simulink model "Bachelor_PanizEilkhani"  (R2020b)
settings: Solver=VariableStepAuto  StartTime=0.0  StopTime=80  RelTol=1e-3
libraries: simulink x3
settings Model: Creator=takro  LastModifiedBy=takro

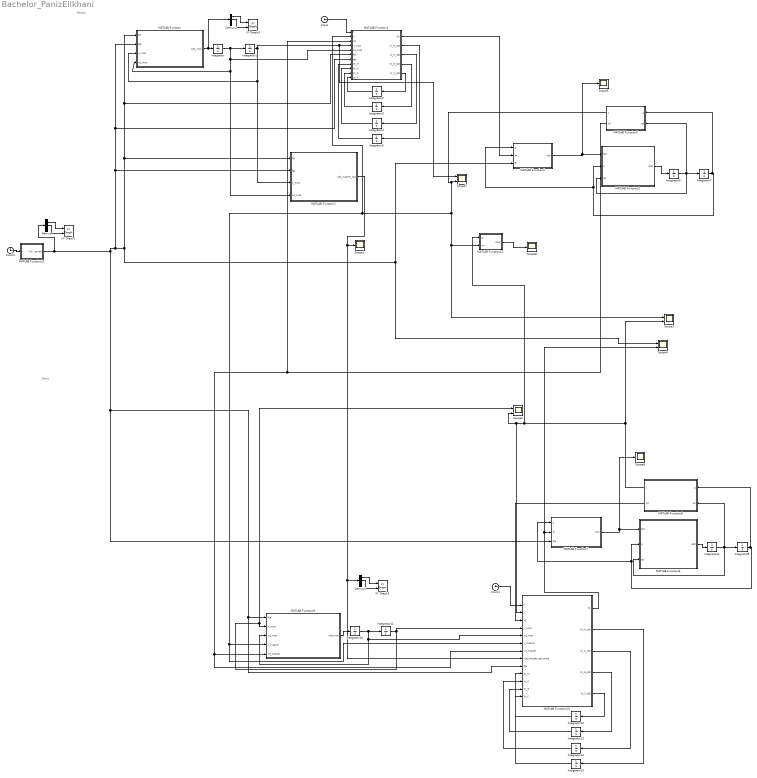
== system Bachelor_PanizEilkhani ==
  note: Master
  note: ُSlave
  Clock : Clock
  Clock1 : Clock
  Clock2 : Clock
  Demux : Demux  Outputs=3
  Demux1 : Demux  Outputs=3
  Demux2 : Demux  Outputs=3
  Integrator{,1,10..11} (4 alike) : Integrator  InitialCondition=[1 1 1]'*0
  Integrator{2..3,12..13} (4 alike) : Integrator  InitialCondition=ones(3, 3)
  Integrator{4..5,14..15} (4 alike) : Integrator  InitialCondition=ones(9, 3)
  Integrator{6..9} (4 alike) : Integrator  InitialCondition=[1 1 1]*0
  MATLAB Function : MATLAB Function  TreatAsAtomicUnit=on
  MATLAB Function1 : MATLAB Function  TreatAsAtomicUnit=on
  MATLAB Function10 : MATLAB Function  TreatAsAtomicUnit=on
  MATLAB Function11 : MATLAB Function  TreatAsAtomicUnit=on
  MATLAB Function12 : MATLAB Function  TreatAsAtomicUnit=on
  MATLAB Function2 : MATLAB Function  TreatAsAtomicUnit=on
  MATLAB Function3 : MATLAB Function  TreatAsAtomicUnit=on
  MATLAB Function4 : MATLAB Function  TreatAsAtomicUnit=on
  MATLAB Function5 : MATLAB Function  TreatAsAtomicUnit=on
  MATLAB Function6 : MATLAB Function  TreatAsAtomicUnit=on
  MATLAB Function7 : MATLAB Function  TreatAsAtomicUnit=on
  MATLAB Function8 : MATLAB Function  TreatAsAtomicUnit=on
  MATLAB Function9 : MATLAB Function  TreatAsAtomicUnit=on
  Scope{1,5..6,8} (4 alike) : Scope
  Scope{2..4,7} (4 alike) : Scope  NumInputPorts=2
  XY Graph1 : simulink/Sinks/XY Graph  xmin=-20  xmax=20  ymin=-20  ymax=20  st=0
  XY Graph2 : simulink/Sinks/XY Graph  xmin=-20  xmax=20  ymin=-20  ymax=20  st=0
  XY Graph3 : simulink/Sinks/XY Graph  xmin=-20  xmax=20  ymin=-20  ymax=20  st=0
  wires:
  Clock/1 -> MATLAB Function1/1(t)
  Integrator5/1 -> MATLAB Function1/8(W_M)
  MATLAB Function1/5(W_F_dot) -> Integrator2/1
  Integrator2/1 -> MATLAB Function1/11(W_F)
  MATLAB Function1/2(W_M_dot) -> Integrator5/1
  MATLAB Function1/3(W_C_dot) -> Integrator4/1
  Integrator/1 -> Integrator1/1, MATLAB Function1/5(xd_mod), MATLAB Function2/4(xd_mod), MATLAB Function/4(xd_mod)
  MATLAB Function1/4(W_G_dot) -> Integrator3/1
  Integrator4/1 -> MATLAB Function1/9(W_C)
  Integrator1/1 -> Scope7/1, MATLAB Function1/4(x_mod), MATLAB Function2/3(x_mod), MATLAB Function/3(x_mod)
  Integrator3/1 -> MATLAB Function1/10(W_G)
  MATLAB Function4/1(taw) -> Scope5/1, MATLAB Function3/1(taw)
  MATLAB Function3/1(qdd) -> Integrator6/1
  Integrator6/1 -> MATLAB Function5/2(qd), MATLAB Function3/3(qd), Integrator7/1
  MATLAB Function1/1(fm) -> MATLAB Function4/2(fm)
  Integrator7/1 -> MATLAB Function5/1(q), MATLAB Function4/1(q), MATLAB Function3/2(q)
  Integrator8/1 -> MATLAB Function8/2(qd), MATLAB Function6/3(qd), Integrator9/1
  MATLAB Function6/1(qdd) -> Integrator8/1
  Integrator9/1 -> MATLAB Function8/1(q), MATLAB Function7/1(q), MATLAB Function6/2(q)
  MATLAB Function7/1(taw) -> Scope6/1, MATLAB Function6/1(taw)
  MATLAB Function5/2(xd) -> MATLAB Function9/5(xd_master), MATLAB Function10/7(xd_master), MATLAB Function1/3(xd)
  Integrator12/1 -> MATLAB Function10/13(W_F)
  MATLAB Function10/2(W_M_dot) -> Integrator15/1
  MATLAB Function10/1(fs) -> Scope4/2, MATLAB Function7/2(fs)
  MATLAB Function10/5(W_F_dot) -> Integrator12/1
  Integrator11/1 -> MATLAB Function10/4(x_mod), Scope2/1, MATLAB Function9/2(x_mod)
  MATLAB Function8/2(xd) -> MATLAB Function10/3(xd)
  MATLAB Function2/1(xdd_master_hat) -> Demux1/1, MATLAB Function10/8(xdd_master_estimate), Scope1/1
  Integrator13/1 -> MATLAB Function10/12(W_G)
  Integrator15/1 -> MATLAB Function10/10(W_M)
  MATLAB Function10/3(W_C_dot) -> Integrator14/1
  Clock1/1 -> MATLAB Function10/1(t)
  Integrator14/1 -> MATLAB Function10/11(W_C)
  Integrator10/1 -> MATLAB Function10/5(xd_mod), MATLAB Function9/3(xd_mod), Integrator11/1
  MATLAB Function5/1(x) -> Scope7/2, MATLAB Function12/2(xm), Scope3/1, MATLAB Function10/6(x_master), MATLAB Function9/4(x_master), MATLAB Function1/2(x)
  MATLAB Function11/1(Xm_desired) -> Demux/1, MATLAB Function7/3(fpa), MATLAB Function10/9(fpa), MATLAB Function9/1(fpa), Scope4/1, MATLAB Function4/3(fh), MATLAB Function/1(fth), MATLAB Function1/6(fth), MATLAB Function2/1(fth), MATLAB Function/2(fpa), MATLAB Function1/7(fpa), MATLAB Function2/2(fpa)
  MATLAB Function9/1(xdd_mod) -> Integrator10/1
  MATLAB Function10/4(W_G_dot) -> Integrator13/1
  Clock2/1 -> MATLAB Function11/1(t)
  Demux/1 -> XY Graph2/1
  Demux/2 -> XY Graph2/2
  Demux1/2 -> XY Graph1/2
  Demux1/1 -> XY Graph1/1
  MATLAB Function8/1(x) -> Scope3/2, MATLAB Function12/1(xs), MATLAB Function10/2(x), Scope2/2
  MATLAB Function12/1(out3) -> Scope8/1
  Demux2/1 -> XY Graph3/1
  MATLAB Function/1(xdd_mod) -> Demux2/1, Integrator/1
  Demux2/2 -> XY Graph3/2

== matlab function Bachelor_PanizEilkhani/MATLAB Function10 ==
  data: t input; x input; fs output; xd input; x_mod input; xd_mod input; x_master input; xd_master input; xdd_master_estimate input; fpa input; W_M input; W_C input; W_G input; W_M_dot output; W_C_dot output; W_G_dot output; W_F_dot output; W_F input
function [fs, W_M_dot, W_C_dot, W_G_dot, W_F_dot] = slave_controller(t, x, xd, x_mod, xd_mod, x_master, xd_master, xdd_master_estimate, fpa, W_M, W_C, W_G, W_F)

landa1 = 1;
landa2 = 3;
landa3 = 0;
kp = 1;
m = eye(3)*15;
c = eye(3)*2500;
k = eye(3)*14000;
invm = inv(m);

fn = 5;
    
zz = [1; sin(fn*t); sin(2*fn*t)];
Z_M = [zz zeros(3, 2) ; zeros(3, 1) zz zeros(3, 1); zeros(3, 2) zz];
Z_C = Z_M;
Z_G = zz; % note G is not like above ones
Z_F = zz; % note F is not like above ones

M_hat = W_M'*Z_M;
C_hat = W_C'*Z_C;
G_hat = W_G'*Z_G;
F_hat = W_F'*Z_F;

Q_M = eye(9)*100;
Q_C = eye(9)*100;
Q_G = eye(3)*100; % note the dimention
Q_F = eye(3)*100; % note the dimention

R = kp*xdd_master_estimate - (invm*c)*(xd-kp*xd_master) - (invm*k)*(x - kp*x_master) + invm*(-fpa) + (landa3^2)*(x-x_mod);
S = (xd-xd_mod) + landa1*(x-x_mod);

W_M_dot = -pinv(Q_M)*Z_M*R*S';
W_C_dot = -pinv(Q_C)*Z_C*xd*S';
W_G_dot = -pinv(Q_G)*Z_G*S';
W_F_dot = -pinv(Q_F)*Z_F*S';


% M_hat = eye(3)*1;
% C_hat = eye(3)*1;
% G_hat = [1 1 1]';
% F_hat = [1 1 1]';

eta = 0.001;
fs = M_hat*R + C_hat*xd + G_hat + F_hat + fpa - eta*sign(S);

end

== matlab function Bachelor_PanizEilkhani/MATLAB Function9 ==
  data: xdd_mod output; fpa input; x_mod input; xd_mod input; x_master input; xd_master input
function xdd_mod = slave_impedance_model(fpa, x_mod, xd_mod, x_master, xd_master)

kp = 1;
m = eye(3)*30;
c = eye(3)*2500;
k = eye(3)*12000;


xdd_mod = pinv(m)*(-fpa - c*(xd_mod - kp*xd_master) - k*(x_mod - kp*x_master));

end

== matlab function Bachelor_PanizEilkhani/MATLAB Function1 ==
  data: t input; x input; fm output; xd input; x_mod input; xd_mod input; fth input; fpa input; W_M input; W_C input; W_G input; W_M_dot output; W_C_dot output; W_G_dot output; W_F_dot output; W_F input
function [fm, W_M_dot, W_C_dot, W_G_dot, W_F_dot] = master_controller(t, x, xd, x_mod, xd_mod, fth, fpa, W_M, W_C, W_G, W_F)

kf = 2;
landa1 = 1;
landa2 = 3;
landa3 = 0;
m = eye(3)*0.2;
c = eye(3)*3;
k = eye(3)*9;
invm = inv(m);

fn = 5;
    
zz = [1; sin(fn*t); sin(2*fn*t)];
Z_M = [zz zeros(3, 2) ; zeros(3, 1) zz zeros(3, 1); zeros(3, 2) zz];
Z_C = Z_M;
Z_G = zz; % note G is not like above ones
Z_F = zz; % note F is not like above ones

M_hat = W_M'*Z_M;
C_hat = W_C'*Z_C;
G_hat = W_G'*Z_G;
F_hat = W_F'*Z_F;

Q_M = eye(9)*1;
Q_C = eye(9)*1;
Q_G = eye(3)*1; % note the dimention
Q_F = eye(3)*1; % note the dimention

R = -(invm*c)*xd - (invm*k)*x + invm*(fth-kf*fpa) + (landa3^2)*(x - x_mod);
S = (xd - xd_mod) + landa1*(x - x_mod);

W_M_dot = -pinv(Q_M)*Z_M*R*S';
W_C_dot = -pinv(Q_C)*Z_C*xd*S';
W_G_dot = -pinv(Q_G)*Z_G*S';
W_F_dot = -pinv(Q_F)*Z_F*S';


% M_hat = eye(3)*1;
% C_hat = eye(3)*1;
% G_hat = [1 1 1]';
% F_hat = [1 1 1]';

fm = M_hat*(R) + C_hat*xd + G_hat + F_hat - fth;


end

== matlab function Bachelor_PanizEilkhani/MATLAB Function2 ==
  data: fth input; xdd_master_hat output; fpa input; x_mod input; xd_mod input
function xdd_master_hat = master_acc_estimator(fth, fpa, x_mod, xd_mod)

kf = 2;
m = eye(3)*0.2;
c = eye(3)*3;
k = eye(3)*9;



invm = inv(m);
xdd_master_hat = invm*(fth-kf*fpa) - invm*c*xd_mod - invm*k*x_mod;



end

== matlab function Bachelor_PanizEilkhani/MATLAB Function3 ==
  data: taw input; q input; qdd output; qd input
function qdd = system(taw, q, qd)

q1 = q(1);
q2 = q(2);
q3 = q(3);

qd1 = qd(1);
qd2 = qd(2);
qd3 = qd(3);

d11=0.00166;
d22=0.018+0.00212*cos(q1)^2+0.0016*sin(q1)^2;
d33=0.0096+0.00426*sin(q2)^2+cos(q2)^2*(0.0141+0.00212*sin(q1)^2+0.0016*cos(q1)^2);
D=[d11,0,0;0,d22,0;0,0,d33];
c12=0.00052*cos(q1)*sin(q1)*qd1;
c13=-0.00052*cos(q2)^2*cos(q1)*sin(q1)*qd3;
c21=1/2*(-0.00104*cos(q1)*sin(q1))*qd2;
c22=1/2*(-0.00104*cos(q1)*sin(q1))*qd1;
c31=1/2*(0.00104*cos(q2)^2*cos(q1)*sin(q1)*qd3);
c23=(-0.5*(0.00852*cos(q2)*sin(q2)-2*sin(q2)*(0.0141+0.00212*sin(q1)^2+0.0016*cos(q1)^2)*cos(q2)))*qd3;
c32=(0.5*(0.00852*sin(q2)*cos(q2)-2*cos(q2)*(0.0141+0.00212*sin(q1)^2+0.0016*cos(q1)^2)*sin(q2)))*qd3;
c33=(0.5*(0.00852*sin(q2)*cos(q2)-2*cos(q2)*sin(q2)*(0.0141+0.00212*sin(q1)^2+0.0016*cos(q1)^2)*(0.00104*cos(q2)^2*cos(q1)*sin(q1)))*qd1);
C=[0,c12,c13;c21,c22,c23;c31,c32,c33];
g11=0.15680*sin(q3)*cos(q1)-0.15680*cos(q3)*sin(q2)*sin(q1);
g21=0.15680*cos(q3)*cos(q2)*cos(q1)-0.479318*cos(q3)*sin(q2);
g31=0.15680*cos(q3)*sin(q1)-0.15680*sin(q3)*sin(q2)*cos(q2);
G=[g11;g21;g31];
Fq = [0.08147*qd1; 0.09058*qd2; 0.127*qd3]*0.05; % random


qdd = pinv(D)*(taw-C*q-G-Fq);


end

== matlab function Bachelor_PanizEilkhani/MATLAB Function6 ==
  data: taw input; q input; qdd output; qd input
function qdd = system(taw, q, qd)

q1 = q(1);
q2 = q(2);
q3 = q(3);

qd1 = qd(1);
qd2 = qd(2);
qd3 = qd(3);

d11=0.00166;
d22=0.018+0.00212*cos(q1)^2+0.0016*sin(q1)^2;
d33=0.0096+0.00426*sin(q2)^2+cos(q2)^2*(0.0141+0.00212*sin(q1)^2+0.0016*cos(q1)^2);
D=[d11,0,0;0,d22,0;0,0,d33];
c12=0.00052*cos(q1)*sin(q1)*qd1;
c13=-0.00052*cos(q2)^2*cos(q1)*sin(q1)*qd3;
c21=1/2*(-0.00104*cos(q1)*sin(q1))*qd2;
c22=1/2*(-0.00104*cos(q1)*sin(q1))*qd1;
c31=1/2*(0.00104*cos(q2)^2*cos(q1)*sin(q1)*qd3);
c23=(-0.5*(0.00852*cos(q2)*sin(q2)-2*sin(q2)*(0.0141+0.00212*sin(q1)^2+0.0016*cos(q1)^2)*cos(q2)))*qd3;
c32=(0.5*(0.00852*sin(q2)*cos(q2)-2*cos(q2)*(0.0141+0.00212*sin(q1)^2+0.0016*cos(q1)^2)*sin(q2)))*qd3;
c33=(0.5*(0.00852*sin(q2)*cos(q2)-2*cos(q2)*sin(q2)*(0.0141+0.00212*sin(q1)^2+0.0016*cos(q1)^2)*(0.00104*cos(q2)^2*cos(q1)*sin(q1)))*qd1);
C=[0,c12,c13;c21,c22,c23;c31,c32,c33];
g11=0.15680*sin(q3)*cos(q1)-0.15680*cos(q3)*sin(q2)*sin(q1);
g21=0.15680*cos(q3)*cos(q2)*cos(q1)-0.479318*cos(q3)*sin(q2);
g31=0.15680*cos(q3)*sin(q1)-0.15680*sin(q3)*sin(q2)*cos(q2);
G=[g11;g21;g31];
Fq = [0.08147*qd1; 0.09058*qd2; 0.127*qd3]*0.05; % random


qdd = pinv(D)*(taw-C*q-G-Fq);

== matlab function Bachelor_PanizEilkhani/MATLAB Function4 ==
  data: q input; fm input; taw output; fh input
function taw = inverse_kinematic(q, fm, fh)

q1 = q(1);
q2 = q(2);
q3 = q(3);

J = eye(3);

taw = J'*(fm + fh);


end

== matlab function Bachelor_PanizEilkhani/MATLAB Function5 ==
  data: q input; x output; qd input; xd output
function [x, xd] = kinematic(q, qd)

q1 = q(1);
q2 = q(2);
q3 = q(3);

J = eye(3);



x = J*q;
xd = J*qd;

end

== matlab function Bachelor_PanizEilkhani/MATLAB Function11 ==
  data: t input; Xm_desired output
function Xm_desired  = fcn(t)
x=10;
y=10;
z=0;

if t<10
x=t;
y=0;
z=0;
end 

if t<20 && t>10
x=10-t;
y=0;
z=0;
end

if t<30 && t>20
x=0;
y=20-t;
z=0;
end

if t<40 && t>30
x=0;
y=40-t;
z=0;
end

if t<50 && t>40
x=50-t;
y=50-t;
z=0;
end

if t<60 && t>50
x=-60+t;
y=60-t;
z=0;
end

if t<70 && t>60
x=70-t;
y=-70+t;
z=0;
end

if t<80 && t>70
x=-80+t;
y=-80+t;
z=0;
end

Xm_desired = [x; y; z];

== matlab function Bachelor_PanizEilkhani/MATLAB Function ==
  data: fth input; xdd_mod output; fpa input; x_mod input; xd_mod input
function xdd_mod = master_impedance_model(fth, fpa, x_mod, xd_mod)

kf = 2;
m = eye(3)*0.2;
c = eye(3)*3;
k = eye(3)*9;


xdd_mod = pinv(m)*(fth - kf*fpa - c*xd_mod - k*x_mod);

end

== matlab function Bachelor_PanizEilkhani/MATLAB Function12 ==
  data: xs input; out3 output; xm input
function out3  = fcn(xs , xm)

out3 = [xs(3),xm(3)];

== matlab function Bachelor_PanizEilkhani/MATLAB Function7 ==
  data: q input; fs input; taw output; fpa input
function taw = inverse_kinematic(q, fs, fpa)

q1 = q(1);
q2 = q(2);
q3 = q(3);

J = eye(3);

taw = J'*(fs + fpa);


end

== matlab function Bachelor_PanizEilkhani/MATLAB Function8 ==
  data: q input; x output; qd input; xd output
function [x, xd] = kinematic(q, qd)

q1 = q(1);
q2 = q(2);
q3 = q(3);

J = eye(3);


x = J*q;
xd = J*qd;

end
